simulink model "long_quad"  (R2017a)
settings: Solver=FixedStepAuto  StartTime=0.0  StopTime=20.0  FixedStep=1e-3  RelTol=1e-3  EnableMultiTasking=on
values from neighbouring files (symbols this model uses):
  C_Dl_quad = 0.05    [init_quad.m]
  C_Dq_quad = 0.5    [init_quad.m]
  g = 9.81    [init_quad.m]
undefined symbols (not defined in the file or in its folder): d_m_quad, J_quad, m_quad, max_sum_force
libraries: simulink_extras x2
settings Model: Creator=gislefh  LastModifiedBy=jljoberg
settings DataIOCC: LimitDataPoints=on  SaveFormat=Array
settings OptimizationCC: LifeSpan=inf
settings DebuggingCC: SFUnexpectedBacktrackingDiag=warning  SFNoUnconditionalDefaultTransitionDiag=warning  SFExecutionAtInitializationDiag=none
settings HardwareCC: ProdBitPerPointer=32  ProdBitPerSizeT=32  ProdBitPerPtrDiffT=32  ProdLargestAtomicFloat=None  ProdIntDivRoundTo=Undefined  ProdEndianess=Unspecified  ProdWordSize=32  ProdHWDeviceType=32-bit Generic
settings ModelReferenceCC: PropagateSignalLabelsOutOfModel=off
settings GRTTargetCC: TargetLangStandard=C89/C90 (ANSI)  GeneratePreprocessorConditionals=Disable all
settings ConfigComp: CovMetricSettings=dw  CovHtmlReporting=on  CovSaveCumulativeToWorkspaceVar=on  CovSaveSingleToWorkspaceVar=on  CovExternalEMLEnable=off

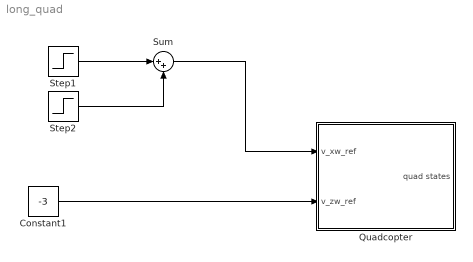
== system long_quad ==
  Constant1 : Constant  Value=-3
  Quadcopter : Subsystem
  Step1 : Step  Time=5  After=17  SampleTime=0
  Step2 : Step  Time=14  After=-5  SampleTime=0
  Sum : Sum  Inputs=|++
  wires:
  Step1/1 -> Sum/1
  Step2/1 -> Sum/2
  Constant1/1 -> Quadcopter/2(v_zw_ref)
  Sum/1 -> Quadcopter/1(v_xw_ref)

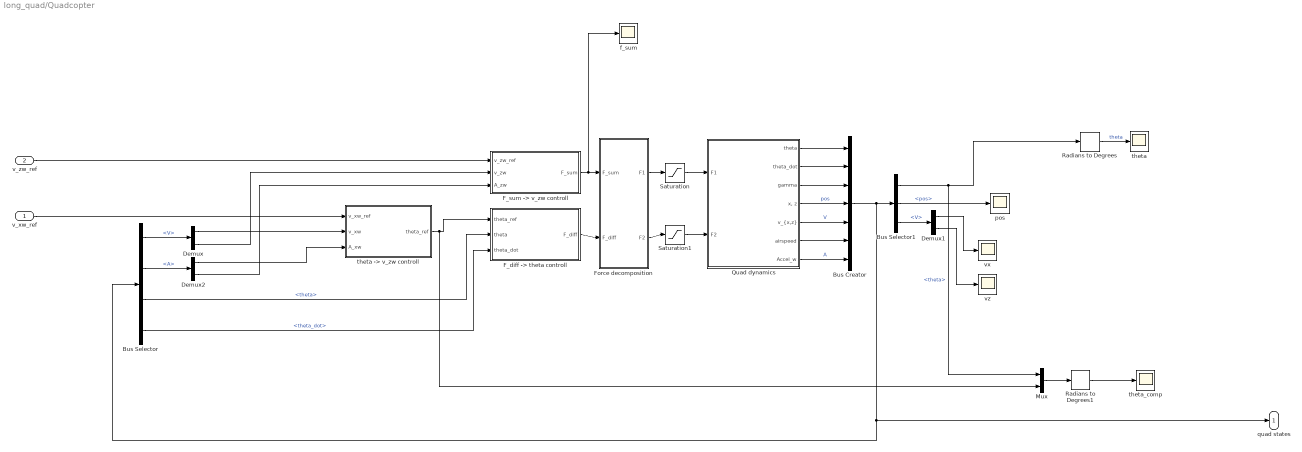
== system long_quad/Quadcopter ==
  v_xw_ref : Inport
  v_zw_ref : Inport  Port=2
  Bus Creator : BusCreator  Inputs=7
  Bus Selector : BusSelector  OutputSignals=V,A,theta,theta_dot
  Bus Selector1 : BusSelector  OutputSignals=theta,pos,V
  Demux : Demux  Outputs=2
  Demux1 : Demux  Outputs=2
  Demux2 : Demux  Outputs=2
  "F_diff -> theta controll" : Subsystem
  "F_sum -> v_zw controll" : Subsystem
  Force decomposition : Subsystem
  Mux : Mux  Inputs=2
  Quad dynamics : Subsystem
  Radians to Degrees : simulink_extras/Transformations/Radians to Degrees
  Radians to Degrees1 : simulink_extras/Transformations/Radians to Degrees
  Saturation : Saturate  UpperLimit=max_sum_force/2  LowerLimit=-max_sum_force/2
  Saturation1 : Saturate  UpperLimit=max_sum_force/2  LowerLimit=-max_sum_force/2
  f_sum : Scope
  "pos " : Scope
  theta : Scope
  "theta -> v_zw controll" : Subsystem
  theta_comp : Scope
  vx : Scope
  "vz " : Scope
  quad states : Outport
  wires:
  Force decomposition/2(F2) -> Saturation1/1
  Bus Selector/4 -> "F_diff -> theta controll"/3(theta_dot)  "<theta_dot>"
  Bus Selector/3 -> "F_diff -> theta controll"/2(theta)  "<theta>"
  Quad dynamics/7(Accel_w) -> Bus Creator/7  "A"
  Saturation1/1 -> Quad dynamics/2(F2)
  Saturation/1 -> Quad dynamics/1(F1)
  Radians to Degrees/1 -> theta/1  "theta"
  Demux1/2 -> "vz "/1
  Quad dynamics/6(airspeed) -> Bus Creator/6
  v_zw_ref/1 -> "F_sum -> v_zw controll"/1(v_zw_ref)
  "F_sum -> v_zw controll"/1(F_sum) -> f_sum/1, Force decomposition/1(F_sum)
  Bus Creator/1 -> Bus Selector/1, quad states/1, Bus Selector1/1
  Bus Selector/1 -> Demux/1  "<V>"
  Quad dynamics/2(theta_dot) -> Bus Creator/2
  Bus Selector/2 -> Demux2/1  "<A>"
  Demux/1 -> "theta -> v_zw controll"/2(v_xw)
  Demux2/1 -> "theta -> v_zw controll"/3(A_xw)
  Bus Selector1/2 -> "pos "/1  "<pos>"
  Quad dynamics/3(gamma) -> Bus Creator/3
  Quad dynamics/4("x, z") -> Bus Creator/4  "pos"
  Bus Selector1/3 -> Demux1/1  "<V>"
  Quad dynamics/1(theta) -> Bus Creator/1
  Radians to Degrees1/1 -> theta_comp/1
  Quad dynamics/5("v_{x,z}") -> Bus Creator/5  "V"
  Bus Selector1/1 -> Mux/1, Radians to Degrees/1  "<theta>"
  Demux/2 -> "F_sum -> v_zw controll"/2(v_zw)
  "theta -> v_zw controll"/1(theta_ref) -> Mux/2, "F_diff -> theta controll"/1(theta_ref)
  Force decomposition/1(F1) -> Saturation/1
  Mux/1 -> Radians to Degrees1/1
  Demux2/2 -> "F_sum -> v_zw controll"/3(A_zw)
  Demux1/1 -> vx/1
  "F_diff -> theta controll"/1(F_diff) -> Force decomposition/2(F_diff)
  v_xw_ref/1 -> "theta -> v_zw controll"/1(v_xw_ref)

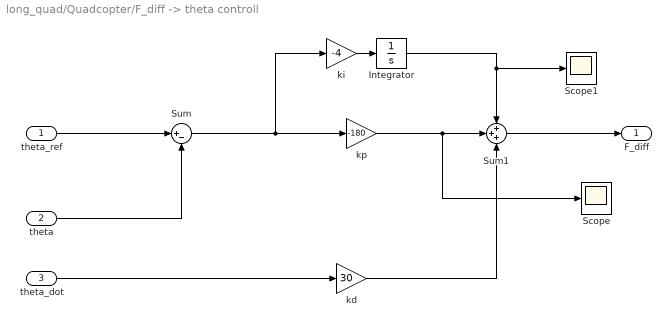
== system long_quad/Quadcopter/F_diff -> theta controll ==
  theta_ref : Inport
  theta : Inport  Port=2
  theta_dot : Inport  Port=3
  Integrator : Integrator
  Scope : Scope
  Scope1 : Scope
  Sum : Sum  Inputs=|+-
  Sum1 : Sum  Inputs=+++
  kd : Gain  Gain=30
  ki : Gain  Gain=-4
  kp : Gain  Gain=-180
  F_diff : Outport
  wires:
  kp/1 -> Scope/1, Sum1/2
  Sum1/1 -> F_diff/1
  Sum/1 -> kp/1, ki/1
  ki/1 -> Integrator/1
  theta/1 -> Sum/2
  theta_ref/1 -> Sum/1
  theta_dot/1 -> kd/1
  kd/1 -> Sum1/3
  Integrator/1 -> Scope1/1, Sum1/1

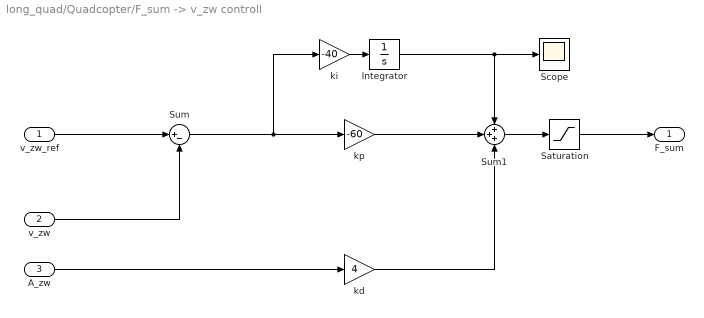
== system long_quad/Quadcopter/F_sum -> v_zw controll ==
  v_zw_ref : Inport
  v_zw : Inport  Port=2
  A_zw : Inport  Port=3
  Integrator : Integrator  LimitOutput=on  UpperSaturationLimit=max_sum_force  LowerSaturationLimit=-max_sum_force
  Saturation : Saturate  UpperLimit=max_sum_force  LowerLimit=-max_sum_force
  Scope : Scope
  Sum : Sum  Inputs=|+-
  Sum1 : Sum  Inputs=+++
  kd : Gain  Gain=4
  ki : Gain  Gain=-40
  kp : Gain  Gain=-60
  F_sum : Outport
  wires:
  v_zw_ref/1 -> Sum/1
  v_zw/1 -> Sum/2
  ki/1 -> Integrator/1
  Sum/1 -> ki/1, kp/1
  Integrator/1 -> Scope/1, Sum1/1
  Sum1/1 -> Saturation/1
  kp/1 -> Sum1/2
  A_zw/1 -> kd/1
  kd/1 -> Sum1/3
  Saturation/1 -> F_sum/1

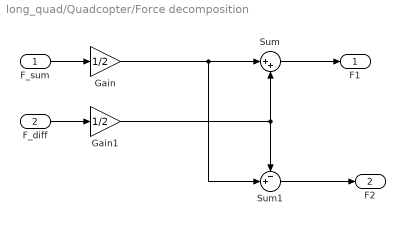
== system long_quad/Quadcopter/Force decomposition ==
  F_sum : Inport
  F_diff : Inport  Port=2
  Gain : Gain  Gain=1/2
  Gain1 : Gain  Gain=1/2
  Sum : Sum  Inputs=|++
  Sum1 : Sum  Inputs=-+|
  F1 : Outport
  F2 : Outport  Port=2
  wires:
  Sum/1 -> F1/1
  Sum1/1 -> F2/1
  Gain/1 -> Sum1/2, Sum/1
  F_diff/1 -> Gain1/1
  Gain1/1 -> Sum1/1, Sum/2
  F_sum/1 -> Gain/1

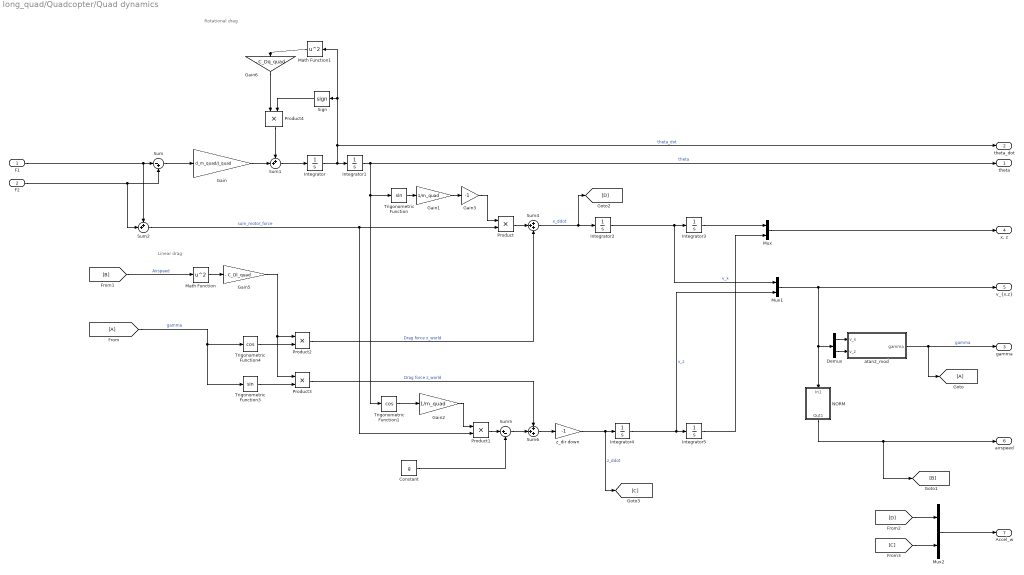
== system long_quad/Quadcopter/Quad dynamics ==
  note: Rotational drag
  note: Linear drag
  F1 : Inport
  F2 : Inport  Port=2
  Constant : Constant  Value=g
  Demux : Demux  Outputs=2
  Gain : Gain  Gain=d_m_quad/J_quad
  Gain1 : Gain  Gain=1/m_quad
  Gain2 : Gain  Gain=1/m_quad
  Gain3 : Gain  Gain=-1
  Gain5 : Gain  Gain=- C_Dl_quad
  Gain6 : Gain  Gain=- C_Dq_quad
  Integrator{,2..5} (5 alike) : Integrator
  Integrator1 : Integrator  InitialCondition=5*deg2rad
  Math Function : Math  Operator=square  SaturateOnIntegerOverflow=on
  Math Function1 : Math  Operator=square  SaturateOnIntegerOverflow=on
  Mux : Mux  Inputs=2
  Mux1 : Mux  Inputs=2
  Mux2 : Mux  Inputs=2
  NORM : Subsystem
  Product{,1..4} (5 alike) : Product
  Sign : Signum
  Sum : Sum  Inputs=|-+
  Sum1 : Sum  Inputs=++|
  Sum2 : Sum  Inputs=++|
  Sum4 : Sum  Inputs=+++
  Sum5 : Sum  Inputs=|+-
  Sum6 : Sum  Inputs=+++
  Trigonometric Function : Trigonometry
  Trigonometric Function1 : Trigonometry  Operator=cos
  Trigonometric Function3 : Trigonometry
  Trigonometric Function4 : Trigonometry  Operator=cos
  atan2_mod : MATLAB Function  TreatAsAtomicUnit=on
  z_dir down : Gain  Gain=-1
  theta : Outport
  theta_dot : Outport  Port=2
  gamma : Outport  Port=3
  "x, z" : Outport  Port=4
  "v_{x,z}" : Outport  Port=5
  airspeed : Outport  Port=6
  Accel_w : Outport  Port=7
  wires:
  Integrator/1 -> theta_dot/1, Sign/1, Math Function1/1, Integrator1/1  "theta_dot"
  Integrator1/1 -> Trigonometric Function1/1, Trigonometric Function/1, theta/1  "theta"
  F1/1 -> Sum2/1, Sum/1
  F2/1 -> Sum2/2, Sum/2
  Sum/1 -> Gain/1
  Gain/1 -> Sum1/2
  Sum1/1 -> Integrator/1
  Integrator2/1 -> Mux1/1, Integrator3/1  "v_x"
  Trigonometric Function/1 -> Gain1/1
  Gain1/1 -> Gain3/1
  Sum2/1 -> Product/2, Product1/2  "sum_motor_force"
  Product/1 -> Sum4/2
  Sum4/1 -> [D], Integrator2/1  "x_ddot"
  Integrator4/1 -> Mux1/2, Integrator5/1  "v_z"
  Integrator5/1 -> Mux/2
  Gain2/1 -> Product1/1
  Sum5/1 -> Sum6/2
  Sum6/1 -> z_dir down/1
  Trigonometric Function1/1 -> Gain2/1
  Mux/1 -> "x, z"/1
  Integrator3/1 -> Mux/1
  Mux1/1 -> NORM/1(In1), Demux/1, "v_{x,z}"/1
  NORM/1(Out1) -> [B], airspeed/1
  Demux/1 -> atan2_mod/1(v_x)
  Demux/2 -> atan2_mod/2(v_z)
  atan2_mod/1(gamma) -> [A], gamma/1  "gamma"
  [A] -> Trigonometric Function3/1, Trigonometric Function4/1  "gamma"
  [B] -> Math Function/1  "Airspeed"
  Math Function/1 -> Gain5/1
  Gain5/1 -> Product3/1, Product2/1
  Trigonometric Function4/1 -> Product2/2
  Trigonometric Function3/1 -> Product3/2
  Math Function1/1 -> Gain6/1
  Product3/1 -> Sum6/1  "Drag force z_world"
  Product2/1 -> Sum4/3  "Drag force x_world"
  Gain6/1 -> Product4/1
  Sign/1 -> Product4/2
  Product4/1 -> Sum1/1
  Product1/1 -> Sum5/1
  Constant/1 -> Sum5/2
  z_dir down/1 -> [C], Integrator4/1  "z_ddot"
  [C] -> Mux2/2
  [D] -> Mux2/1
  Mux2/1 -> Accel_w/1
  Gain3/1 -> Product/1

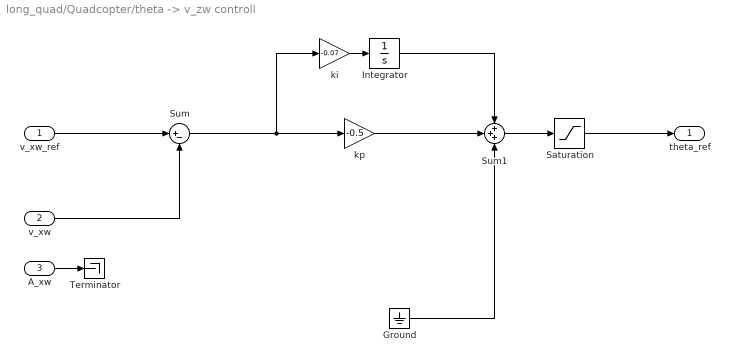
== system long_quad/Quadcopter/theta -> v_zw controll ==
  v_xw_ref : Inport
  v_xw : Inport  Port=2
  A_xw : Inport  Port=3
  Ground : Ground
  Integrator : Integrator  LimitOutput=on  UpperSaturationLimit=80*deg2rad  LowerSaturationLimit=-80*deg2rad
  Saturation : Saturate  UpperLimit=80*deg2rad  LowerLimit=-80*deg2rad
  Sum : Sum  Inputs=|+-
  Sum1 : Sum  Inputs=+++
  Terminator : Terminator
  ki : Gain  Gain=-0.07
  kp : Gain  Gain=-0.5
  theta_ref : Outport
  wires:
  kp/1 -> Sum1/2
  Sum1/1 -> Saturation/1
  Integrator/1 -> Sum1/1
  ki/1 -> Integrator/1
  v_xw/1 -> Sum/2
  v_xw_ref/1 -> Sum/1
  Saturation/1 -> theta_ref/1
  Sum/1 -> ki/1, kp/1
  A_xw/1 -> Terminator/1
  Ground/1 -> Sum1/3

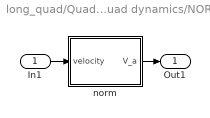
== system long_quad/Quadcopter/Quad dynamics/NORM ==
  In1 : Inport
  norm : MATLAB Function  TreatAsAtomicUnit=on
  Out1 : Outport
  wires:
  norm/1(V_a) -> Out1/1
  In1/1 -> norm/1(velocity)

== matlab function long_quad/Quadcopter/Quad dynamics/atan2_mod ==
  data: v_x input; gamma output; v_z input
function gamma = atan2_mod(v_x,v_z)

if v_x == 0
    gamma = 90;
    if v_z == 0
        gamma = 0;
    end
else
    gamma = atan2(v_z,v_x);
end
gamma = -gamma;
end

== matlab function long_quad/Quadcopter/Quad dynamics/NORM/norm ==
  data: velocity input; V_a output
function V_a = norm(velocity)
V_a = norm(velocity);
